simulink model "s_function_from_em"  (R2015a)
settings: Solver=ode45  StartTime=0.0  StopTime=10.0  RelTol=1e-3
libraries: simulink x4
settings Model: CovSFcnEnable=off  Creator=teme  LastModifiedBy=teme
settings DataIOCC: SaveFormat=Structure  SaveOutput=off  SaveTime=off
settings OptimizationCC: InlineParams=on

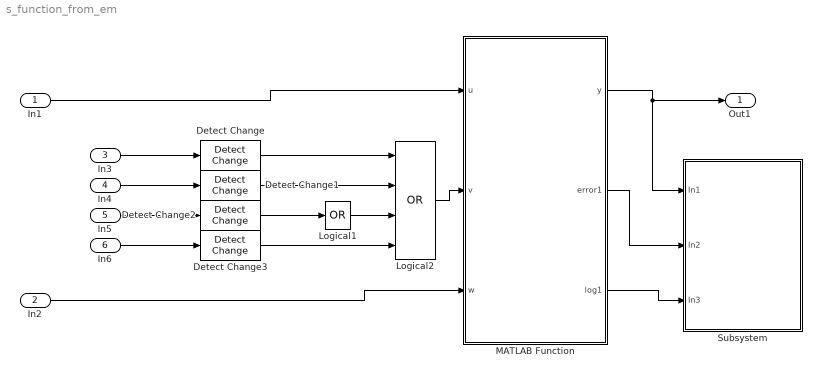
== system s_function_from_em ==
  In1 : Inport  OutDataTypeStr=double  PortDimensions=1  BusOutputAsStruct=on
  In2 : Inport  Port=2  OutDataTypeStr=double  PortDimensions=1
  In3 : Inport  Port=3  OutDataTypeStr=double  PortDimensions=1  BusOutputAsStruct=on
  In4 : Inport  Port=4  OutDataTypeStr=double  PortDimensions=1  BusOutputAsStruct=on
  In5 : Inport  Port=5  OutDataTypeStr=double  PortDimensions=1  BusOutputAsStruct=on
  In6 : Inport  Port=6  OutDataTypeStr=double  PortDimensions=1  BusOutputAsStruct=on
  Detect Change{,1..3} (4 alike) : simulink/Logic and Bit Operations/Detect Change  vinit=0  InputProcessing=Inherited  OutDataTypeStr=boolean
  Logical1 : Logic  Operator=OR  Inputs=1  AllPortsSameDT=off  OutDataTypeStr=boolean
  Logical2 : Logic  Operator=OR  Inputs=4  AllPortsSameDT=off  OutDataTypeStr=boolean
  MATLAB Function : Subsystem
      mask help: Simulink:masks:GenSFuncDesc_MD
      mask Help: eval('feval(''rtwprivate'',''rtwhelpview'',''rtw_sfcn_block'')');
  Subsystem : Subsystem  TreatAsAtomicUnit=on
  Out1 : Outport
  wires:
  In1/1 -> MATLAB Function/1(u)
  Logical2/1 -> MATLAB Function/2(v)
  Logical1/1 -> Logical2/3
  Detect Change/1 -> Logical2/1
  Detect Change1/1 -> Logical2/2
  Detect Change2/1 -> Logical1/1
  Detect Change3/1 -> Logical2/4
  In4/1 -> Detect Change1/1
  In3/1 -> Detect Change/1
  In5/1 -> Detect Change2/1
  In6/1 -> Detect Change3/1
  In2/1 -> MATLAB Function/3(w)
  MATLAB Function/1(y) -> Subsystem/1(In1), Out1/1
  MATLAB Function/2(error1) -> Subsystem/2(In2)
  MATLAB Function/3(log1) -> Subsystem/3(In3)

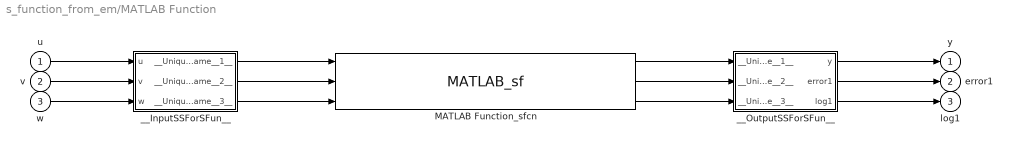
== system s_function_from_em/MATLAB Function ==
  u : Inport
  v : Inport  Port=2
  w : Inport  Port=3
  MATLAB Function_sfcn : S-Function  FunctionName=MATLAB_sf  SFunctionModules=""  mask{rtw_sf_name=MATLAB_sf, showVar=off}
      mask prompts: rtw_sf_name "Simulink:masks:GenSFuncName_MP"; showVar "Simulink:masks:GenSFuncShowModuleList_MP"
      mask help: Simulink:masks:GenSFuncDesc_MD
      mask init:
      | displist = '';
      | if ~strcmp(get_param(gcb, 'FunctionName'), rtw_sf_name);
      |   set_param(gcb, 'FunctionName', rtw_sf_name);
      | end
      | % Check if we are generating code
      | rtw_mode = false;
      | if strcmpi(get_param(bdroot(gcb),'SimulationStatus'),'Initializing')
      | 	rtw_mode = strcmpi(get_param(bdroot(gcb),'BuildingRTWCode'),'on') && ...
      | 		~strcmpi(get_param(bdroot(gcb),'TargetStyle'),'SimulationTarget');
      | end
      | if showVar || rtw_mode
      | 	if exist('rtwsfunc') == 2 | exist('rtwsfunc') == 6
      | 		tmplist = rtwsfunc(rtw_sf_name,gcb);
      | 		tmplist = DAStudio.message('Simulink:masks:GenSFuncListOfModules_IC', tmplist);
      | 	elseif showVar
      | 		tmplist1 = DAStudio.message('Simulink:masks:GenSFuncListOfModules_IC', '');
      |         tmplist2 = DAStudio.message('Simulink:masks:GenSFuncNotLicensed_IC');
      |         tmplist = [tmplist1 tmplist2];
      |  	end
      | end
      | if showVar
      |   displist = tmplist;
      | end
      settings: CopyFcn=|
      | if ~strcmp(get_param(gcb,'Linkstatus'),'none') && ...
      | ~strcmp(get_param(gcb,'Linkstatus'),'implicit')
      |   set_param(gcb,'LinkStatus','none');
      | end
      mask Help: eval('feval(''rtwprivate'',''rtwhelpview'',''rtw_sfcn_block'')');
      mask Display:
      | port_label('input',1,'u');
      | port_label('input',2,'v');
      | port_label('input',3,'w');
      | port_label('output',1,'y');
      | port_label('output',2,'error1');
      | port_label('output',3,'log1');
  __InputSSForSFun__ : Subsystem
  __OutputSSForSFun__ : Subsystem
  y : Outport
  error1 : Outport  Port=2
  log1 : Outport  Port=3
  wires:
  u/1 -> __InputSSForSFun__/1(u)
  v/1 -> __InputSSForSFun__/2(v)
  w/1 -> __InputSSForSFun__/3(w)
  __InputSSForSFun__/1(__UniqueOutportName__1__) -> MATLAB Function_sfcn/1
  __InputSSForSFun__/2(__UniqueOutportName__2__) -> MATLAB Function_sfcn/2
  __InputSSForSFun__/3(__UniqueOutportName__3__) -> MATLAB Function_sfcn/3
  MATLAB Function_sfcn/1 -> __OutputSSForSFun__/1(__UniqueInportName__1__)
  MATLAB Function_sfcn/2 -> __OutputSSForSFun__/2(__UniqueInportName__2__)
  MATLAB Function_sfcn/3 -> __OutputSSForSFun__/3(__UniqueInportName__3__)
  __OutputSSForSFun__/1(y) -> y/1
  __OutputSSForSFun__/2(error1) -> error1/1
  __OutputSSForSFun__/3(log1) -> log1/1

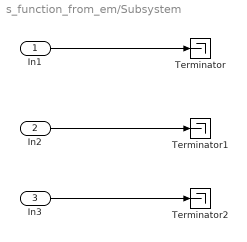
== system s_function_from_em/Subsystem ==
  In1 : Inport
  In2 : Inport  Port=2
  In3 : Inport  Port=3
  Terminator : Terminator
  Terminator1 : Terminator
  Terminator2 : Terminator
  wires:
  In1/1 -> Terminator/1
  In2/1 -> Terminator1/1
  In3/1 -> Terminator2/1

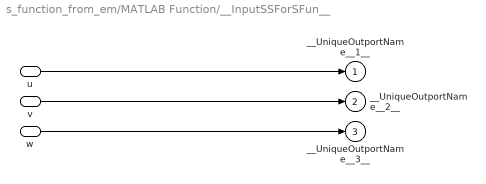
== system s_function_from_em/MATLAB Function/__InputSSForSFun__ ==
  u : Inport
  v : Inport  Port=2
  w : Inport  Port=3
  __UniqueOutportName__1__ : Outport
  __UniqueOutportName__2__ : Outport  Port=2
  __UniqueOutportName__3__ : Outport  Port=3
  wires:
  u/1 -> __UniqueOutportName__1__/1
  v/1 -> __UniqueOutportName__2__/1
  w/1 -> __UniqueOutportName__3__/1

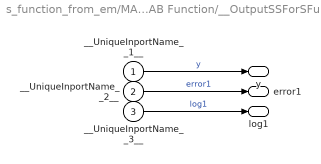
== system s_function_from_em/MATLAB Function/__OutputSSForSFun__ ==
  __UniqueInportName__1__ : Inport
  __UniqueInportName__2__ : Inport  Port=2
  __UniqueInportName__3__ : Inport  Port=3
  y : Outport
  error1 : Outport  Port=2
  log1 : Outport  Port=3
  wires:
  __UniqueInportName__1__/1 -> y/1  "y"
  __UniqueInportName__2__/1 -> error1/1  "error1"
  __UniqueInportName__3__/1 -> log1/1  "log1"
